simulink model "HDLHeaderGen"  (R2024a)
settings: Solver=FixedStepDiscrete  StartTime=0.0  StopTime=stopTime  RelTol=1e-3
values from neighbouring files (symbols this model uses):
  fs = 1    [testHeaderGen.m]
libraries: dspsrcs4 x5, HDL_ieee_8021513 x2, whdlutilities x1
settings Model: DataTypeOverride=Off  Creator=cotti  LastModifiedBy=cotti
settings OptimizationCC: BlockReduction=off  ConditionallyExecuteInputs=off  DefaultParameterBehavior=Inlined  InheritOutputTypeSmallerThanSingle=on
settings DebuggingCC: AlgebraicLoopMsg=error  ArtificialAlgebraicLoopMsg=error  SingleTaskRateTransMsg=error  UnconnectedInputMsg=warning  UnconnectedOutputMsg=warning  UnconnectedLineMsg=warning
settings HardwareCC: ProdBitPerPointer=32  ProdBitPerSizeT=32  ProdBitPerPtrDiffT=32  ProdLargestAtomicFloat=None  ProdIntDivRoundTo=Undefined  ProdEndianess=Unspecified  ProdWordSize=32  ProdHWDeviceType=ASIC/FPGA->ASIC/FPGA  TargetBitPerLong=64  TargetBitPerPointer=64  TargetBitPerSizeT=64  TargetBitPerPtrDiffT=64  TargetLongLongMode=on  TargetIntDivRoundTo=Zero  TargetEndianess=LittleEndian  TargetWordSize=64  TargetHWDeviceType=Custom Processor->MATLAB Host Computer  ProdEqTarget=off

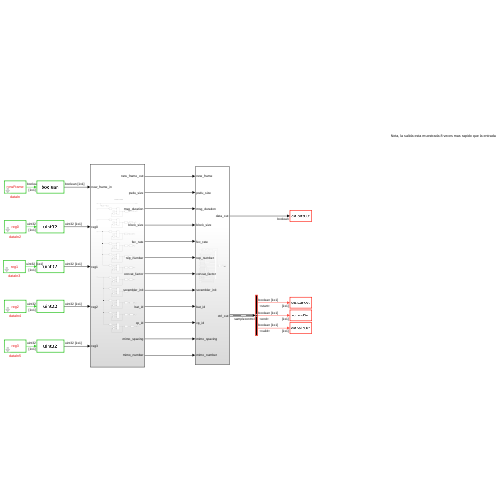
[thumbnail: Simulink's stored preview of the top-level diagram]
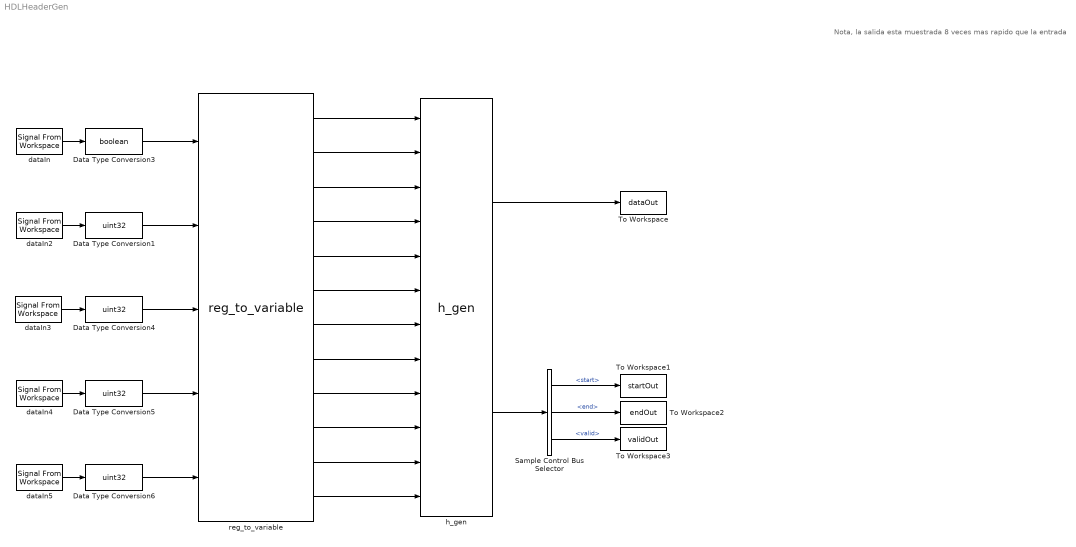
== system HDLHeaderGen ==
  note: Nota, la salida esta muestrada 8 veces mas rapido que la entrada
  Data Type Conversion{1,4..6} (4 alike) : DataTypeConversion  OutDataTypeStr=uint32  SaturateOnIntegerOverflow=off  RndMeth=Floor
  Data Type Conversion3 : DataTypeConversion  OutDataTypeStr=boolean  SaturateOnIntegerOverflow=off  RndMeth=Floor
  Sample Control Bus Selector : whdlutilities/Sample Control Bus Selector  OutputSignals=start,end,valid
  To Workspace : ToWorkspace  VariableName=dataOut  SampleTime=1/(8*fs)
      settings: Save2DSignal=2-D array (concatenate along first dimension)
  To Workspace1 : ToWorkspace  VariableName=startOut  SampleTime=1/(8*fs)
      settings: Save2DSignal=2-D array (concatenate along first dimension)
  To Workspace2 : ToWorkspace  VariableName=endOut  SampleTime=1/(8*fs)
      settings: Save2DSignal=2-D array (concatenate along first dimension)
  To Workspace3 : ToWorkspace  VariableName=validOut  SampleTime=1/(8*fs)
      settings: Save2DSignal=2-D array (concatenate along first dimension)
  dataIn : dspsrcs4/Signal From Workspace  X=newFrame  Ts=1/fs  nsamps=1  OutputAfterFinalValue=Setting to zero  ignoreOrWarnInputAndFrameLengths=off  OutputFrames=off
  dataIn2 : dspsrcs4/Signal From Workspace  X=reg0  Ts=1/fs  nsamps=1  OutputAfterFinalValue=Holding final value  ignoreOrWarnInputAndFrameLengths=off  OutputFrames=off
  dataIn3 : dspsrcs4/Signal From Workspace  X=reg1  Ts=1/fs  nsamps=1  OutputAfterFinalValue=Holding final value  ignoreOrWarnInputAndFrameLengths=off  OutputFrames=off
  dataIn4 : dspsrcs4/Signal From Workspace  X=reg2  Ts=1/fs  nsamps=1  OutputAfterFinalValue=Holding final value  ignoreOrWarnInputAndFrameLengths=off  OutputFrames=off
  dataIn5 : dspsrcs4/Signal From Workspace  X=reg3  Ts=1/fs  nsamps=1  OutputAfterFinalValue=Holding final value  ignoreOrWarnInputAndFrameLengths=off  OutputFrames=off
  h_gen : HDL_ieee_8021513/h_gen  SystemSampleTime=-1  VariantActivationTime=update diagram  AllowFlexibleInterface=on  Latency=0  AutoFrameSizeCalculation=off
      settings: SourceProductName=HDL IEEE 8021513
  reg_to_variable : HDL_ieee_8021513/reg_to_variable  SystemSampleTime=-1  VariantActivationTime=update diagram  AllowFlexibleInterface=on  Latency=0  AutoFrameSizeCalculation=off
      settings: SourceProductName=HDL IEEE 8021513
  wires:
  Sample Control Bus Selector/3 -> To Workspace3/1  "<valid>"
  Sample Control Bus Selector/1 -> To Workspace1/1  "<start>"
  h_gen/2 -> Sample Control Bus Selector/1
  h_gen/1 -> To Workspace/1
  reg_to_variable/12 -> h_gen/12
  reg_to_variable/11 -> h_gen/11
  reg_to_variable/10 -> h_gen/10
  reg_to_variable/9 -> h_gen/9
  reg_to_variable/6 -> h_gen/6
  reg_to_variable/5 -> h_gen/5
  reg_to_variable/4 -> h_gen/4
  dataIn/1 -> Data Type Conversion3/1
  dataIn2/1 -> Data Type Conversion1/1
  dataIn3/1 -> Data Type Conversion4/1
  reg_to_variable/8 -> h_gen/8
  Data Type Conversion3/1 -> reg_to_variable/1
  reg_to_variable/2 -> h_gen/2
  dataIn4/1 -> Data Type Conversion5/1
  Data Type Conversion1/1 -> reg_to_variable/2
  Sample Control Bus Selector/2 -> To Workspace2/1  "<end>"
  Data Type Conversion5/1 -> reg_to_variable/4
  dataIn5/1 -> Data Type Conversion6/1
  reg_to_variable/1 -> h_gen/1
  Data Type Conversion4/1 -> reg_to_variable/3
  reg_to_variable/7 -> h_gen/7
  Data Type Conversion6/1 -> reg_to_variable/5
  reg_to_variable/3 -> h_gen/3
